simulink model "final_project_dscrt"  (R2019b)
settings: Solver=FixedStepAuto  StartTime=0.0  StopTime=10.0  FixedStep=0.01  RelTol=1e-3
undefined symbols (not defined in the file or in its folder): DiscIntNeverNeededParam
libraries: simulink x1
settings Model: Creator=Mertcan  LastModifiedBy=Mertcan

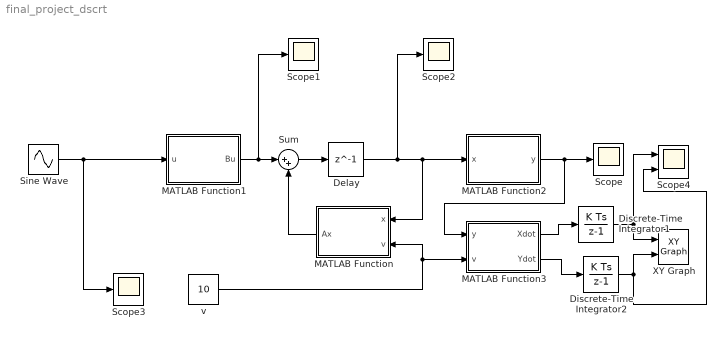
== system final_project_dscrt ==
  Delay : Delay  DelayLength=1  SampleTime=0.01
  Discrete-Time Integrator1 : DiscreteIntegrator  SampleTime=0.01  ICPrevOutput=DiscIntNeverNeededParam  ICPrevScaledInput=DiscIntNeverNeededParam
  Discrete-Time Integrator2 : DiscreteIntegrator  SampleTime=0.01  ICPrevOutput=DiscIntNeverNeededParam  ICPrevScaledInput=DiscIntNeverNeededParam
  MATLAB Function : MATLAB Function  TreatAsAtomicUnit=on
  MATLAB Function1 : MATLAB Function  TreatAsAtomicUnit=on
  MATLAB Function2 : MATLAB Function  TreatAsAtomicUnit=on
  MATLAB Function3 : MATLAB Function  TreatAsAtomicUnit=on
  Scope{,1..3} (4 alike) : Scope
  Scope4 : Scope  NumInputPorts=2
  Sine Wave : Sin  Amplitude=0.07  SampleTime=0.01
  Sum : Sum  Inputs=|++
  XY Graph : simulink/Sinks/XY Graph  xmin=-1  xmax=100  ymin=-10  ymax=30  st=-1
  v : Constant  Value=10
  wires:
  MATLAB Function/1(Ax) -> Sum/2
  MATLAB Function1/1(Bu) -> Scope1/1, Sum/1
  Sum/1 -> Delay/1
  Sine Wave/1 -> Scope3/1, MATLAB Function1/1(u)
  v/1 -> MATLAB Function3/2(v), MATLAB Function/2(v)
  MATLAB Function2/1(y) -> MATLAB Function3/1(y), Scope/1
  Discrete-Time Integrator1/1 -> Scope4/1, XY Graph/1
  Discrete-Time Integrator2/1 -> Scope4/2, XY Graph/2
  MATLAB Function3/1(Xdot) -> Discrete-Time Integrator1/1
  MATLAB Function3/2(Ydot) -> Discrete-Time Integrator2/1
  Delay/1 -> Scope2/1, MATLAB Function2/1(x), MATLAB Function/1(x)

== matlab function final_project_dscrt/MATLAB Function1 ==
  data: u input; Bu output
function Bu = Bmat(u)

% m = 1350; % kg
% lf = 1.016; % m
% Iz = 4000; % kg.m^2
% Cf = 87594; % N/rad

% dt = 0.1
% B = [0.204160750073782
%     3.22429376254482
%     0.0952067310058050
%     1.74510127293309];

% dt = 0.01

B = [0.00308538121733195
    0.601722163601119
    0.00109699431148174
    0.217836958427102];

Bu = B*u;

== matlab function final_project_dscrt/MATLAB Function ==
  data: x input; Ax output; v input
function Ax = Amat(x,v)

% m = 1350; % kg
% lf = 1.016; % m
% lr = 1.562; % m
% Iz = 4000; % kg.m^2
% Cf = 87594; % N/rad
% Cr = 87594; % N/rad

% dt = 0.1
% A = [1,0.0554395351293068,0,-0.0167590342351909
%     0,0.260529237543850,0,-0.230564952320616
%     0,0.00310316170359759,1,0.0693857231158054
%     0,0.0426922172359289,0,0.452396031479352];

% dt = 0.01

A = [1,0.00937715121894016,0,-0.000301547085405976
    0,0.877953203322308,0,-0.0582583895552142
    0,5.58355185705388e-05,1,0.00962808646263230
    0,0.0107873282460033,0,0.926433470211531];
    
Ax = A*x;

== matlab function final_project_dscrt/MATLAB Function2 ==
  data: x input; y output
function y = Cmat(x)

C = [1, 0, 0, 0
    0, 0, 1, 0];

y = C*x;

== matlab function final_project_dscrt/MATLAB Function3 ==
  data: y input; Xdot output; v input; Ydot output
function [Xdot, Ydot] = CmatXY(y,v)

ydot = y(1);
phi = y(2);

Ydot = sin(phi)*v+cos(phi)*ydot;
Xdot = cos(phi)*v-sin(phi)*ydot;
